simulink model "full_sim"  (R2025a)
settings: Solver=VariableStepAuto  StartTime=0.0  StopTime=10.0  RelTol=1e-3
undefined symbols (not defined in the file or in its folder): fractalcoef
libraries: commchan3 x2, mspsensorlib x1, dspfdesign x1
settings Model: Creator=prana  LastModifiedBy=prana

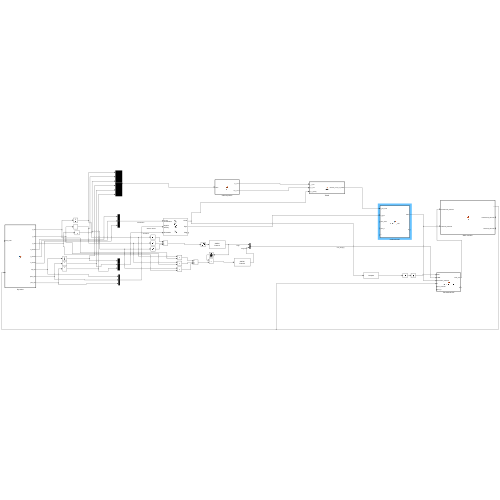
[thumbnail: Simulink's stored preview of the top-level diagram]
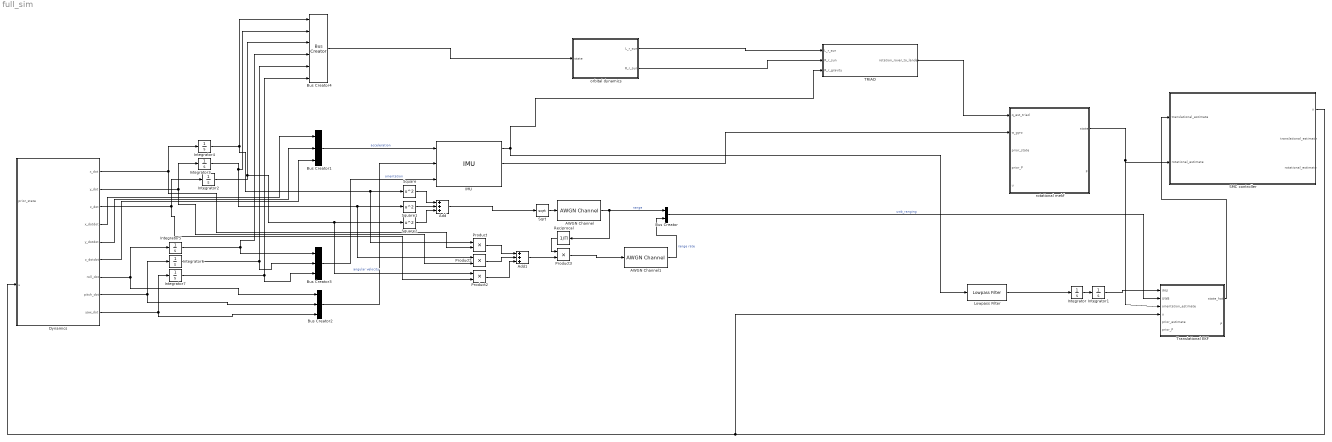
== system full_sim ==
  AWGN Channel : commchan3/AWGN Channel  LegacyMode=off  NoiseMethod="Signal to noise ratio  (SNR)"  noiseMode="Signal to noise ratio  (SNR)"  EbNo=10  EsNo=10  SNR=3  BitsPerSymbol=1  SignalPower=1  SpecifySymbolPeriod=off  SamplesPerSymbol=1  SymbolPeriod=1  VarianceSource=Parameter  Variance=1  RandomStream=Global stream  Seed=67  SimulateUsing=Code generation
  AWGN Channel1 : commchan3/AWGN Channel  LegacyMode=off  NoiseMethod="Signal to noise ratio  (SNR)"  noiseMode="Signal to noise ratio  (SNR)"  EbNo=10  EsNo=10  SNR=3  BitsPerSymbol=1  SignalPower=1  SpecifySymbolPeriod=off  SamplesPerSymbol=1  SymbolPeriod=1  VarianceSource=Parameter  Variance=1  RandomStream=Global stream  Seed=67  SimulateUsing=Code generation
  Add : Sum  Inputs=+++
  Add1 : Sum  Inputs=+++
  Bus Creator : BusCreator  Inputs=2
  Bus Creator1 : BusCreator  Inputs=3
  Bus Creator2 : BusCreator  Inputs=3
  Bus Creator3 : BusCreator  Inputs=3
  Bus Creator4 : BusCreator  Inputs=6
  Dynamics : MATLAB Function  TreatAsAtomicUnit=on
  IMU : mspsensorlib/IMU  DispRefFrame=NED  TemperaturePort=off  Temperature=25  MagneticFieldPort=off  MagneticFieldNED=[ 27.5550, -2.4169, -16.0849 ]  MagneticFieldENU=[ -2.4169, 27.5550, 16.0849 ]  SeedDouble=67  SimulateUsing=Interpreted execution  AccelParamsMeasurementRange=Inf  AccelParamsResolution=0  AccelParamsConstantBias=[ 0, 0, 0 ]  AccelParamsAxesMisalignment=[ 100, 0, 0; 0, 100, 0; 0, 0, 100 ]  AccelParamsNoiseDensity=[ 0, 0, 0 ]  AccelParamsBiasInstability=[ 0, 0, 0 ]  AccelParamsBiasInstabilityNumerator=fractalcoef().Numerator  AccelParamsBiasInstabilityDenominator=fractalcoef().Denominator  AccelParamsRandomWalk=[ 0, 0, 0 ]  AccelParamsNoiseType=double-sided  AccelParamsTemperatureBias=[ 0, 0, 0 ]  AccelParamsTemperatureScaleFactor=[ 0, 0, 0 ]  GyroParamsMeasurementRange=Inf  GyroParamsResolution=0  GyroParamsConstantBias=[ 0, 0, 0 ]  GyroParamsAxesMisalignment=[ 100, 0, 0; 0, 100, 0; 0, 0, 100 ]  GyroParamsAccelerationBias=[ 0, 0, 0 ]  GyroParamsNoiseDensity=[ 0, 0, 0 ]  GyroParamsBiasInstability=[ 0, 0, 0 ]  GyroParamsBiasInstabilityNumerator=fractalcoef().Numerator  GyroParamsBiasInstabilityDenominator=fractalcoef().Denominator  GyroParamsRandomWalk=[ 0, 0, 0 ]  GyroParamsNoiseType=double-sided  GyroParamsTemperatureBias=[ 0, 0, 0 ]  GyroParamsTemperatureScaleFactor=[ 0, 0, 0 ]  MagParamsMeasurementRange=Inf  MagParamsResolution=0  MagParamsConstantBias=[ 0, 0, 0 ]  MagParamsAxesMisalignment=[ 100, 0, 0; 0, 100, 0; 0, 0, 100 ]  MagParamsNoiseDensity=[ 0, 0, 0 ]  MagParamsBiasInstability=[ 0, 0, 0 ]  MagParamsBiasInstabilityNumerator=fractalcoef().Numerator  MagParamsBiasInstabilityDenominator=fractalcoef().Denominator  MagParamsRandomWalk=[ 0, 0, 0 ]  MagParamsNoiseType=double-sided  MagParamsTemperatureBias=[ 0, 0, 0 ]  MagParamsTemperatureScaleFactor=[ 0, 0, 0 ]
  Integrator{,1..7} (8 alike) : Integrator
  Lowpass Filter : dspfdesign/Lowpass Filter  FilterType=FIR  DesignForMinimumOrder=on  FilterOrder=50  PassbandFrequency=0.3628  StopbandFrequency=0.5442  PassbandRipple=0.1  StopbandAttenuation=80  SampleRateMode=Use normalized frequency (0 to 1)  SampleRate=44100  SimulateUsing=Interpreted execution  roundingMode=Floor  coeffsDataTypeStr=fixdt(1,16)
  Product{,1..3} (4 alike) : Product
  Reciprocal : Product  Inputs=/
  SMC controller : MATLAB Function  TreatAsAtomicUnit=on
  Sqrt : Sqrt
  Square : Math  Operator=square
  Square1 : Math  Operator=square
  Square2 : Math  Operator=square
  TRIAD : MATLAB Function  TreatAsAtomicUnit=on
  Translational EKF : MATLAB Function  TreatAsAtomicUnit=on
  orbital dynamics : MATLAB Function  TreatAsAtomicUnit=on
  rotational mekf : MATLAB Function  TreatAsAtomicUnit=on
  wires:
  orbital dynamics/1(L_r_sun) -> TRIAD/1(L_r_sun)
  orbital dynamics/2(R_r_sun) -> TRIAD/2(R_r_sun)
  IMU/1 -> TRIAD/3(R_r_gravity), Lowpass Filter/1
  Integrator/1 -> Integrator1/1
  Integrator1/1 -> Translational EKF/1(IMU)
  Bus Creator/1 -> Translational EKF/2(UWB)  "uwb_ranging"
  Dynamics/4(x_dotdot) -> Bus Creator1/1
  Dynamics/5(y_dotdot) -> Bus Creator1/2
  Dynamics/6(z_dotdot) -> Bus Creator1/3
  Bus Creator1/1 -> IMU/1  "acceleration"
  Dynamics/8(pitch_dot) -> Bus Creator2/2, Integrator6/1
  Dynamics/9(yaw_dot) -> Bus Creator2/3, Integrator7/1
  Dynamics/7(roll_dot) -> Bus Creator2/1, Integrator5/1
  Bus Creator2/1 -> IMU/2  "angular velocity"
  Integrator5/1 -> Bus Creator4/4, Bus Creator3/1
  Integrator6/1 -> Bus Creator3/2, Bus Creator4/5
  Integrator7/1 -> Bus Creator3/3, Bus Creator4/6
  Bus Creator3/1 -> IMU/3  "orientation"
  AWGN Channel/1 -> Reciprocal/1, Bus Creator/1  "range"
  AWGN Channel1/1 -> Bus Creator/2  "range rate"
  Add/1 -> Sqrt/1
  Sqrt/1 -> AWGN Channel/1
  Integrator4/1 -> Product/1, Square/1, Bus Creator4/1
  Integrator3/1 -> Product1/1, Square1/1, Bus Creator4/2
  Integrator2/1 -> Bus Creator4/3, Product2/1, Square2/1
  Square/1 -> Add/1
  Square1/1 -> Add/2
  Square2/1 -> Add/3
  Dynamics/1(x_dot) -> Integrator4/1, Product/2
  Dynamics/2(y_dot) -> Integrator3/1, Product1/2
  Dynamics/3(z_dot) -> Product2/2, Integrator2/1
  Product/1 -> Add1/1
  Product1/1 -> Add1/2
  Product2/1 -> Add1/3
  Reciprocal/1 -> Product3/1
  Add1/1 -> Product3/2
  Product3/1 -> AWGN Channel1/1
  Bus Creator4/1 -> orbital dynamics/1(state)
  IMU/2 -> rotational mekf/2(w_gyro)
  TRIAD/1(rotation_rover_to_lander) -> rotational mekf/1(q_est_triad)
  rotational mekf/1(state) -> Translational EKF/3(orientation_estimate), SMC controller/2("rotational_estimate ")
  Translational EKF/1(state_hat) -> SMC controller/1("translational_estimate ")
  SMC controller/1(u) -> Translational EKF/4(u), Dynamics/2(u)
  Lowpass Filter/1 -> Integrator/1

== matlab function full_sim/TRIAD ==
  data: L_r_sun input; rotation_rover_to_lander output; R_r_sun input; R_r_gravity input
function rotation_rover_to_lander = TRIAD(L_r_sun, R_r_sun, R_r_gravity)

rotation_rover_to_lander = L_r_sun;

end

== matlab function full_sim/orbital dynamics ==
  data: state input; L_r_sun output; R_r_sun output
function [L_r_sun, R_r_sun] = fcn(state)

L_r_sun = 1; 
R_r_sun = 1; 

end

== matlab function full_sim/rotational mekf ==
  data: q_est_triad input; state output; w_gyro input; P output; prior_state input; prior_P input; u input
function [state, P]= rotational_mekf(q_est_triad, w_gyro, prior_state, prior_P, u)
    % nominal state: [q, b] (b is bias)
    % error state: [dq, db] 
    prior_q = prior_state(1:4);
    prior_b = prior_state(5:7);
    rw = 0.085;
    B = 0.2;

    %quaternion propagation (predict step)
    w_corrected = w_gyro - prior_b + [0; 0; rw * (u(1) - u(2)) / B];
    %q_dot = 0.5 * prior_q * quaternion(0, w_corrected(1), w_corrected(2), w_corrected(3));
    %i think the above is right; chat doesn't
    q_dot = 0.5 * quatmultiply(prior_q', quaternion(0, w_corrected(1), w_corrected(2), w_corrected(3)));
    q_pred = prior_q + q_dot * dt;
    q_pred = q_pred / norm(q_pred);
    b_pred = prior_b;
    
    %error state linearized dynamics ?!?!?!?!?!
    %some skew-symmetric matrix representation of a cross product from chat
    w_x = [0, -w_corrected(3), w_corrected(2); 
           w_corrected(3), 0, -w_corrected(1); 
           -w_corrected(2), w_corrected(1), 0];
    F = [-w_x, -eye(3); zeros(3, 6)];
    %phi = eye(6) + F * dt;
    Q_theta = (4.36e-5)^2 * dt * eye(3);
    Q_b = (4e-8)^2 * dt * eye(3);
    P = F * prior_P + prior_P * F' + blkdiag(Q_theta, Q_b);

    %measurement update
    q_err = q_est_triad * conj(q_pred);
    dtheta = 2 * q_err(2:4);
    H = [eye(3), zeros(3, 3)];
    R = 8.7e-3 * eye(3);
    S = H * P * H' + R;
    K = P * H' / S;
    dx = K * dtheta;
    dtheta_corr = dx(1:3);
    db = dx(4:6);
    %i have no idea what this does but chat does!
    function dq = smallAngleQuat(dtheta)

        angle = norm(dtheta);
        
        if angle < 1e-12
            dq = [1 0 0 0];
            return;
        end
        
        axis = dtheta / angle;
        
        dq = axang2quat([axis' angle]);
    end
    dq = smallAngleQuat(dtheta_corr);
    q = quatmultiply(dq, q_pred);
    q = q / norm(q);
    b = b_pred + db;
    P = (eye(6) - K * H) * P;
    state = [q; b];
end

== matlab function full_sim/Translational EKF ==
  data: IMU input; state_hat output; UWB input; orientation_estimate input; u input; prior_estimate input; prior_P input; P output
function [state_hat, P] = translational_ekf(IMU, UWB, orientation_estimate, u, prior_estimate, prior_P)
    %state = [x, y, z, x_dot, y_dot, z_dot]
    %measurement / control unpacking

    x_nminus1 = prior_estimate(1);
    y_nminus1 = prior_estimate(2);
    z_nminus1 = prior_estimate(3);
    x_dot_nminus1 = prior_estimate(4);
    y_dot_nminus1 = prior_estimate(5);
    z_dot_nminus1 = prior_estimate(6);
    rho_nminus1 = norm(prior_estimate(1:3));

    wr = u(1);
    wl = u(2);
    dwr = u(3);
    dwl = u(4);
    v = wr + wl;
    dv = dwr + dwl;

    %roll = orientation_estimate(1);
    pitch = orientation_estimate(2);
    yaw = orientation_estimate(3);

    rw = 0.17/2; %wheel radius, m
    % B = 0.2; %base width, m

    %process noise matrix
    W = diag([0.01; 0.01; 0.05]);

    % MEASUREMENT NOISE TODO
    R = diag(ones(8) * 0.01); 
    
    %predict step
    %state propagation
    state_dot_hat = [cos(yaw) * v; 
                    sin(yaw) * v; 
                    sin(pitch) * v; 
                    cos(yaw) * dv; 
                    sin(yaw) * dv; 
                    sin(pitch) * dv] * rw / 2;
    
    %rw * [cos(yaw) * (wr + wl) / 2; sin(yaw) * (wr + wl) / 2; (wr - wl) / B];
    state_hat_pred = prior_estimate + state_dot_hat * dt;
    
    %covariance propagation
    P_dot = W;
    P_pred = prior_P + P_dot * dt;

    %update step
    alpha = dot(prior_estimate(1:3), prior_estimate(4:6)); 
    H = [eye(6); 
        x_nminus1 / rho_nminus1, y_nminus1 / rho_nminus1, z_nminus1 / rho_nminus1, zeros(1, 3); 
        (x_dot_nminus1 * rho_nminus1 - alpha * x_nminus1 / rho_nminus1) / rho_nminus1^2, ...
        (y_dot_nminus1 * rho_nminus1 - alpha * y_nminus1 / rho_nminus1) / rho_nminus1^2, ...
        (z_dot_nminus1 * rho_nminus1 - alpha * z_nminus1 / rho_nminus1) / rho_nminus1^2, ...
        x_nminus1 / rho_nminus1, y_nminus1 / rho_nminus1, z_nminus1 / rho_nminus1];
    K = P_pred * H' * pinv(H * P_pred * H' + R);
    rho_pred = norm(state_hat_pred(1:3));
    alpha_pred = dot(state_hat_pred(1:3), state_hat_pred(4:6));
    state_hat = state_hat_pred + K * ([IMU; UWB] - [state_hat_pred; rho_pred; alpha_pred / rho_pred]);
    P = (eye(6) - K * H) * P_pred;

end

== matlab function full_sim/Dynamics ==
  data: prior_state input; u input; x_dot output; y_dot output; z_dot output; x_dotdot output; y_dotdot output; z_dotdot output; roll_dot output; pitch_dot output; yaw_dot output
function [x_dot, y_dot, z_dot, x_dotdot, y_dotdot, z_dotdot, roll_dot, pitch_dot, yaw_dot] = fcn(prior_state, u)

y = u;

== matlab function full_sim/SMC controller ==
  data: translational_estimate input; u output; rotational_estimate input; translational_estimate output; rotational_estimate output
function [u, translational_estimate, rotational_estimate] = fcn(translational_estimate, rotational_estimate)

y = u;
